simulink model "Phase_reversal_Jaimin_19_6"  (R2022b)
settings: Solver=ode45  StartTime=0.0  StopTime=10.0  MaxStep=1e-5  MinStep=1e-7  RelTol=1e-6
libraries: spsSeriesRLCBranchLib x3, spsGroundLib x2, spsThreePhaseProgrammableVoltageSourceLib x1, spsThreePhaseVIMeasurementLib x1, spsVoltageMeasurementLib x1, sps_lib x1
settings Model: Creator=E0660158  LastModifiedBy=E0660158

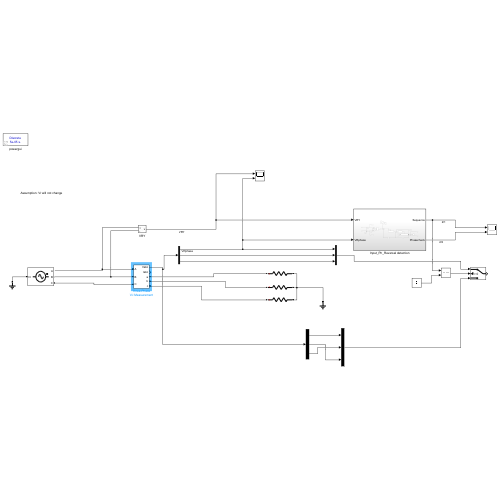
[thumbnail: Simulink's stored preview of the top-level diagram]
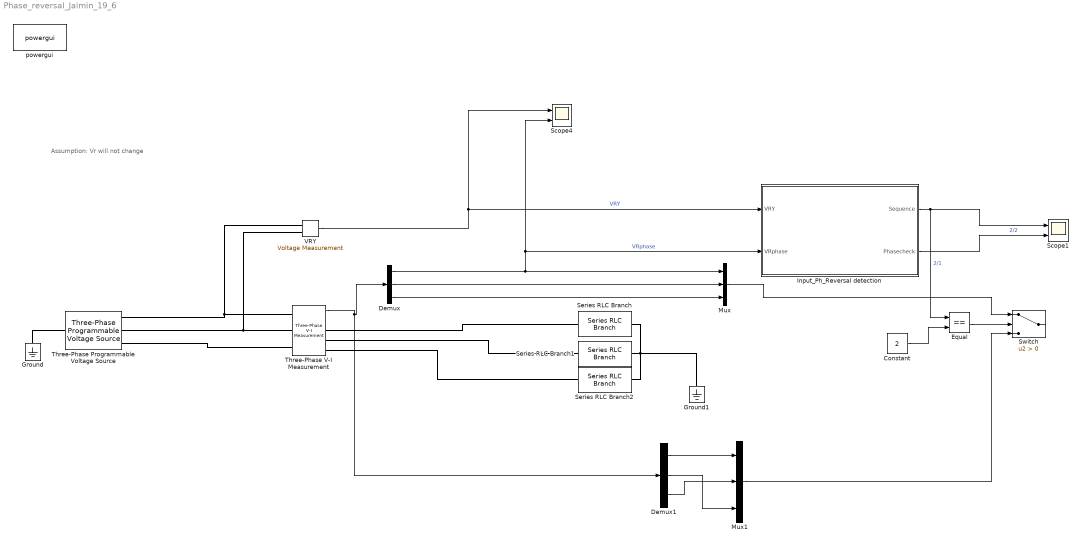
== system Phase_reversal_Jaimin_19_6 ==
  note: Assumption: Vr will not change
  Constant : Constant  Value=2
  Demux : Demux  Outputs=3
  Demux1 : Demux  Outputs=3
  Equal : RelationalOperator  Operator===  OutDataTypeStr=boolean  RndMeth=Simplest  InputSameDT=off
  Ground : spsGroundLib/Ground  LConnTagsString=a
  Ground1 : spsGroundLib/Ground  LConnTagsString=a
  Input_Ph_Reversal detection : Subsystem
  Mux : Mux  Inputs=3
  Mux1 : Mux  Inputs=3
  Scope1 : Scope  NumInputPorts=2
  Scope4 : Scope  NumInputPorts=2
  Series RLC Branch : spsSeriesRLCBranchLib/Series RLC Branch  LConnTagsString=__new0  RConnTagsString=__new0  BranchType=R  Resistance=1  Inductance=1e-3  SetiL0=off  InitialCurrent=0  Capacitance=1e-6  Setx0=off  InitialVoltage=0  Measurements=None
  Series RLC Branch1 : spsSeriesRLCBranchLib/Series RLC Branch  LConnTagsString=__new0  RConnTagsString=__new0  BranchType=R  Resistance=1  Inductance=1e-3  SetiL0=off  InitialCurrent=0  Capacitance=1e-6  Setx0=off  InitialVoltage=0  Measurements=None
  Series RLC Branch2 : spsSeriesRLCBranchLib/Series RLC Branch  LConnTagsString=__new0  RConnTagsString=__new0  BranchType=R  Resistance=1  Inductance=1e-3  SetiL0=off  InitialCurrent=0  Capacitance=1e-6  Setx0=off  InitialVoltage=0  Measurements=None
  Switch : Switch  Criteria=u2 > Threshold  SaturateOnIntegerOverflow=off  InputSameDT=off
  Three-Phase Programmable Voltage Source : spsThreePhaseProgrammableVoltageSourceLib/Three-Phase Programmable Voltage Source  PositiveSequence=[400 0 50]  VariationEntity=None  VariationType=Table of time-amplitude pairs  VariationTypeAlt=Step  VariationStep=0.5  VariationRate=10  VariationMagnitude=0.3  VariationFrequency=2  VariationTiming=[1 2]  VariationPhaseA=off  Amplitudes=[1 0.8 1.2 1.0]  TimeValues=[0 0.1 0.15 0.2]  HarmonicGeneration=off  HarmonicA=[3 0.2 -25 0]  HarmonicB=[2 0.15 35 2]  Timing="[0.05  3]"  BusType=swing  Pref=0  Qref=0  Qmin=-inf  Qmax=inf
  Three-Phase V-I Measurement : spsThreePhaseVIMeasurementLib/Three-Phase V-I Measurement  VoltageMeasurement=phase-to-ground  SetLabelV=off  LabelV=Vabc  Vpu=off  VpuLL=off  CurrentMeasurement=yes  SetLabelI=off  LabelI=Iabc  Ipu=off  Pbase=100e6  Vbase=500e3  OutputType=Complex  PhasorSimulation=off  PSBequivalent=0
  VRY : spsVoltageMeasurementLib/Voltage Measurement  PhasorSimulation=off  OutputType=Complex  PSBequivalent=0
  powergui : sps_lib/powergui  Priority=1  SimulationMode=Discrete  SampleTime=50e-6  frequency=60  Iterations=50  frequencyindice=50  Pbase=100e6  ErrMax=1e-4  UnitsV=kV  UnitsW=MW  buscounter=0  FunctionMessages=off  echomessages=off  EnableUseOfTLC=off  CurrentSourceSwitches=off  DisableSnubberDevices=off  DisableRonSwitches=off  DisableVfSwitches=off  DisplayEquations=off  AutomaticDiscreteSolvers=off  SolverType=Tustin/Backward Euler (TBE)  Interpol=off  ExternalGateDelay=off  methode=off  Ts=100  x0status=blocks  SPID=on  SwTol=0  HookPort=off  NonlinearTolerance=1e-4  nMaxIteration=100  ContinueOnMaxIteration=off  RestoreLinks=warning  ResistiveCurrentMeasurement=off  Frange=[0:2:500]  Ylog=off  Xlog=on  ShowGrid=off  save=off  variable=ZData  structure=0  ZoomFFT=off  StartTime=0.0  cycles=1  DisplayStyle=1  fundamental=60  FreqAxis=off  MaxFrequency=1000  frequencyindicesteady=1  RmsSteady=1  display=off
  wires:
  Demux/1 -> Mux/1, Input_Ph_Reversal detection/2(VRphase), Scope4/2  "VRphase"
  VRY/1 -> Input_Ph_Reversal detection/1(VRY), Scope4/1  "VRY"
  Input_Ph_Reversal detection/1(Sequence) -> Equal/1, Scope1/1  "2/1"
  Input_Ph_Reversal detection/2(Phasecheck) -> Scope1/2  "2/2"
  Constant/1 -> Equal/2
  Equal/1 -> Switch/2
  Mux/1 -> Switch/1
  Demux/2 -> Mux/2
  Demux/3 -> Mux/3
  Three-Phase V-I Measurement/1 -> Demux1/1, Demux/1
  Demux1/1 -> Mux1/1
  Demux1/2 -> Mux1/3
  Demux1/3 -> Mux1/2
  Mux1/1 -> Switch/3
  connections:
  VRY/LConn1 -- Three-Phase Programmable Voltage Source/RConn1 -- Three-Phase V-I Measurement/LConn1
  VRY/LConn2 -- Three-Phase Programmable Voltage Source/RConn2 -- Three-Phase V-I Measurement/LConn2
  Ground/LConn1 -- Three-Phase Programmable Voltage Source/LConn1
  Series RLC Branch/LConn1 -- Three-Phase V-I Measurement/RConn1
  Series RLC Branch1/LConn1 -- Three-Phase V-I Measurement/RConn2
  Series RLC Branch2/LConn1 -- Three-Phase V-I Measurement/RConn3
  Series RLC Branch/RConn1 -- Ground1/LConn1 -- Series RLC Branch1/RConn1 -- Series RLC Branch2/RConn1
  Three-Phase V-I Measurement/LConn3 -- Three-Phase Programmable Voltage Source/RConn3

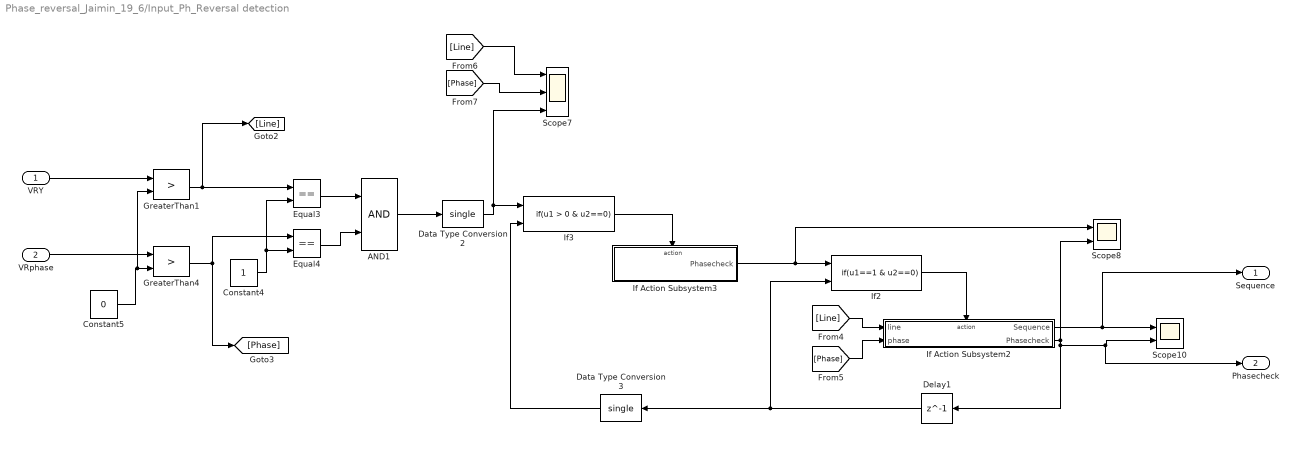
== system Phase_reversal_Jaimin_19_6/Input_Ph_Reversal detection ==
  VRY : Inport
  VRphase : Inport  Port=2
  AND1 : Logic  AllPortsSameDT=off  OutDataTypeStr=boolean
  Constant4 : Constant
  Constant5 : Constant  Value=0
  Data Type Conversion2 : DataTypeConversion  OutDataTypeStr=single  SaturateOnIntegerOverflow=off  RndMeth=Floor
  Data Type Conversion3 : DataTypeConversion  OutDataTypeStr=single  SaturateOnIntegerOverflow=off  RndMeth=Floor
  Delay1 : Delay  DelayLength=1
  Equal3 : RelationalOperator  Operator===  OutDataTypeStr=boolean  RndMeth=Simplest  InputSameDT=off
  Equal4 : RelationalOperator  Operator===  OutDataTypeStr=boolean  RndMeth=Simplest  InputSameDT=off
  GreaterThan1 : RelationalOperator  Operator=>  OutDataTypeStr=boolean  RndMeth=Simplest  InputSameDT=off
  GreaterThan4 : RelationalOperator  Operator=>  OutDataTypeStr=boolean  RndMeth=Simplest  InputSameDT=off
  If Action Subsystem2 : Subsystem  TreatAsAtomicUnit=on
  If Action Subsystem3 : Subsystem  TreatAsAtomicUnit=on
  If2 : If  NumInputs=2  IfExpression=u1==1 & u2==0  ShowElse=off
  If3 : If  NumInputs=2  IfExpression=u1 > 0 & u2==0  ShowElse=off
  Scope10 : Scope  NumInputPorts=2
  Scope7 : Scope  NumInputPorts=3
  Scope8 : Scope  NumInputPorts=2
  Sequence : Outport
  Phasecheck : Outport  Port=2
  wires:
  AND1/1 -> Data Type Conversion2/1
  Data Type Conversion3/1 -> If3/2
  [Phase] -> Scope7/2
  Data Type Conversion2/1 -> If3/1, Scope7/3
  If Action Subsystem2/2(Phasecheck) -> Delay1/1, Phasecheck/1, Scope10/2, Scope8/2
  If Action Subsystem3/1(Phasecheck) -> Scope8/1, If2/1
  [Line] -> Scope7/1
  GreaterThan1/1 -> [Line], Equal3/1
  Equal3/1 -> AND1/1
  [Line] -> If Action Subsystem2/1(line)
  Constant5/1 -> GreaterThan1/2, GreaterThan4/2
  Constant4/1 -> Equal3/2, Equal4/2
  Delay1/1 -> If2/2, Data Type Conversion3/1
  If3/1 -> If Action Subsystem3/Action
  [Phase] -> If Action Subsystem2/2(phase)
  If Action Subsystem2/1(Sequence) -> Sequence/1, Scope10/1
  If2/1 -> If Action Subsystem2/Action
  GreaterThan4/1 -> [Phase], Equal4/1
  Equal4/1 -> AND1/2
  VRY/1 -> GreaterThan1/1
  VRphase/1 -> GreaterThan4/1

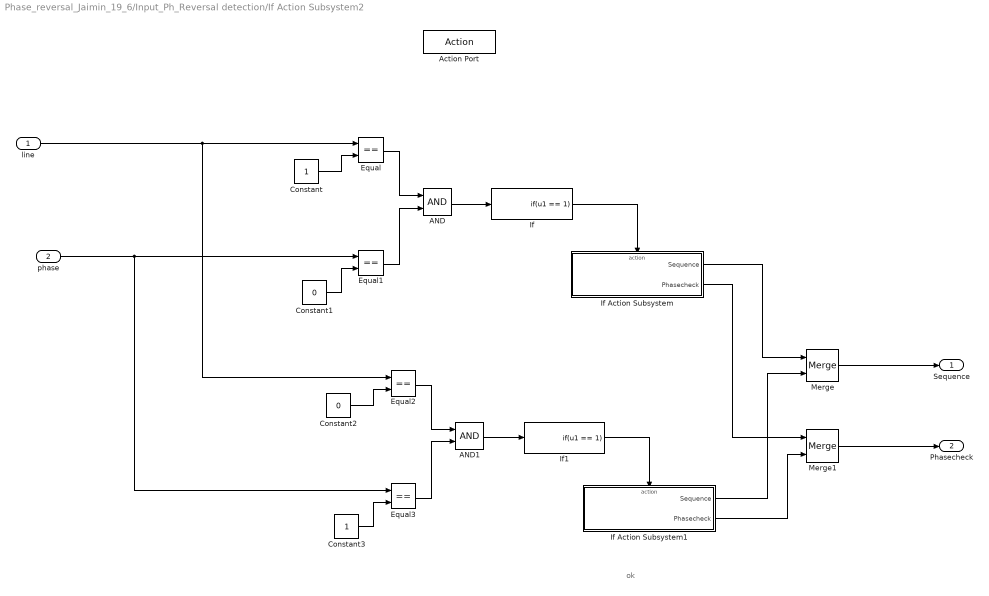
== system Phase_reversal_Jaimin_19_6/Input_Ph_Reversal detection/If Action Subsystem2 ==
  note: ok
  line : Inport
  phase : Inport  Port=2
  Action Port : ActionPort  ActionPortLabel=if(u1==1 & u2==0)
  AND : Logic  AllPortsSameDT=off  OutDataTypeStr=boolean
  AND1 : Logic  AllPortsSameDT=off  OutDataTypeStr=boolean
  Constant : Constant
  Constant1 : Constant  Value=0
  Constant2 : Constant  Value=0
  Constant3 : Constant
  Equal{,1..3} (4 alike) : RelationalOperator  Operator===  OutDataTypeStr=boolean  RndMeth=Simplest  InputSameDT=off
  If : If  IfExpression=u1 == 1  ShowElse=off
  If Action Subsystem : Subsystem  TreatAsAtomicUnit=on
  If Action Subsystem1 : Subsystem  TreatAsAtomicUnit=on
  If1 : If  IfExpression=u1 == 1  ShowElse=off
  Merge : Merge
  Merge1 : Merge
  Sequence : Outport  InitialOutput=[0]
  Phasecheck : Outport  Port=2  InitialOutput=[0]
  wires:
  line/1 -> Equal2/1, Equal/1
  Constant/1 -> Equal/2
  Constant1/1 -> Equal1/2
  Equal1/1 -> AND/2
  Equal/1 -> AND/1
  AND/1 -> If/1
  If/1 -> If Action Subsystem/Action
  If1/1 -> If Action Subsystem1/Action
  AND1/1 -> If1/1
  Equal2/1 -> AND1/1
  Equal3/1 -> AND1/2
  Constant3/1 -> Equal3/2
  phase/1 -> Equal3/1, Equal1/1
  Constant2/1 -> Equal2/2
  If Action Subsystem/1(Sequence) -> Merge/1
  If Action Subsystem1/1(Sequence) -> Merge/2
  Merge/1 -> Sequence/1
  If Action Subsystem/2(Phasecheck) -> Merge1/1
  If Action Subsystem1/2(Phasecheck) -> Merge1/2
  Merge1/1 -> Phasecheck/1

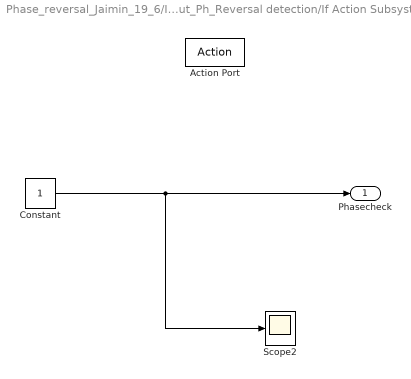
== system Phase_reversal_Jaimin_19_6/Input_Ph_Reversal detection/If Action Subsystem3 ==
  Action Port : ActionPort  ActionPortLabel=if(u1 > 0 & u2==0)
  Constant : Constant
  Scope2 : Scope
  Phasecheck : Outport  InitialOutput=[0]
  wires:
  Constant/1 -> Scope2/1, Phasecheck/1

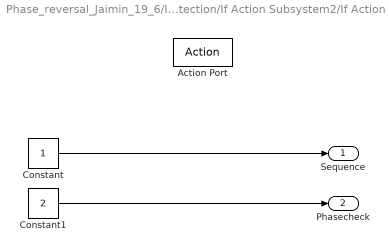
== system Phase_reversal_Jaimin_19_6/Input_Ph_Reversal detection/If Action Subsystem2/If Action Subsystem ==
  Action Port : ActionPort  ActionPortLabel=if(u1 == 1)
  Constant : Constant
  Constant1 : Constant  Value=2
  Sequence : Outport
  Phasecheck : Outport  Port=2
  wires:
  Constant/1 -> Sequence/1
  Constant1/1 -> Phasecheck/1

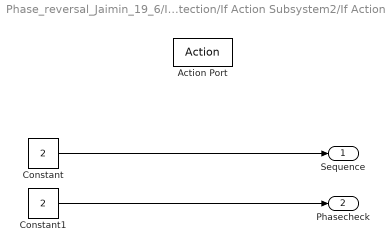
== system Phase_reversal_Jaimin_19_6/Input_Ph_Reversal detection/If Action Subsystem2/If Action Subsystem1 ==
  Action Port : ActionPort  ActionPortLabel=if(u1 == 1)
  Constant : Constant  Value=2
  Constant1 : Constant  Value=2
  Sequence : Outport
  Phasecheck : Outport  Port=2
  wires:
  Constant1/1 -> Phasecheck/1
  Constant/1 -> Sequence/1
